simulink model "pendulotriple"  (R2023b)
settings: Solver=ode15s  StartTime=0.0  StopTime=20  RelTol=1e-3
values from neighbouring files (symbols this model uses):
  BL = 0.00223579    [ILCadaptable.m]    (also in parametros3.m)
  C1 = [1 0 0 0]    [ILCadaptable.m]    (also in parametros3.m = [1 0 0 0 0 0])
  C2 = [0 1 0 0]    [ILCadaptable.m]    (also in parametros3.m = [0 0 1 0 0 0])
  C3 = [0 0 1 0]    [ILCadaptable.m]    (also in parametros3.m = [0 0 0 0 1 0])
  Cv1 = [0 1 0 0 0 0]    [parametros3.m]
  Cv2 = [0 0 0 1 0 0]    [parametros3.m]
  Cv3 = [0 0 0 0 0 1]    [parametros3.m]
  ek1_1 = out.ek1    [ILCadaptable.m]    (also in parametros3.m)
  ek2_1 = out.ek2    [ILCadaptable.m]    (also in parametros3.m)
  ek3_1 = out.ek3    [parametros3.m]
  JL = 0.00040095    [ILCadaptable.m]    (also in parametros3.m)
  KB = 0.23351629    [ILCadaptable.m]    (also in parametros3.m)
  KM = 0.23351629    [ILCadaptable.m]    (also in parametros3.m)
  L1 = 2    [ILCadaptable.m]    (also in parametros3.m)
  L2 = 2    [ILCadaptable.m]    (also in parametros3.m)
  L3 = 2    [ILCadaptable.m]    (also in parametros3.m)
  LC = 0.0015    [ILCadaptable.m]    (also in parametros3.m)
  RC = 3.4    [ILCadaptable.m]    (also in parametros3.m)
  rt = 10    [ILCadaptable.m]    (also in parametros3.m)
libraries: slpidlib x3, simulink x3
settings Model: Creator=LENOVO  LastModifiedBy=LENOVO

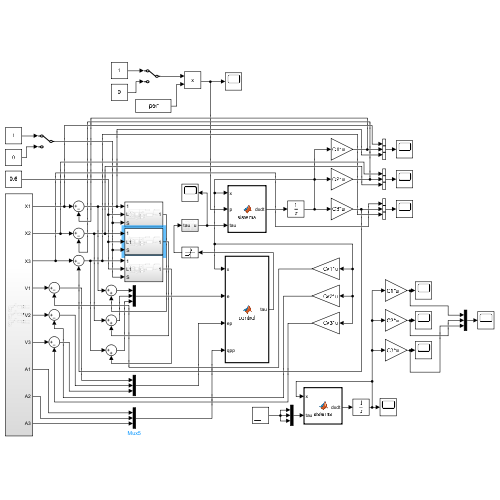
[thumbnail: Simulink's stored preview of the top-level diagram]
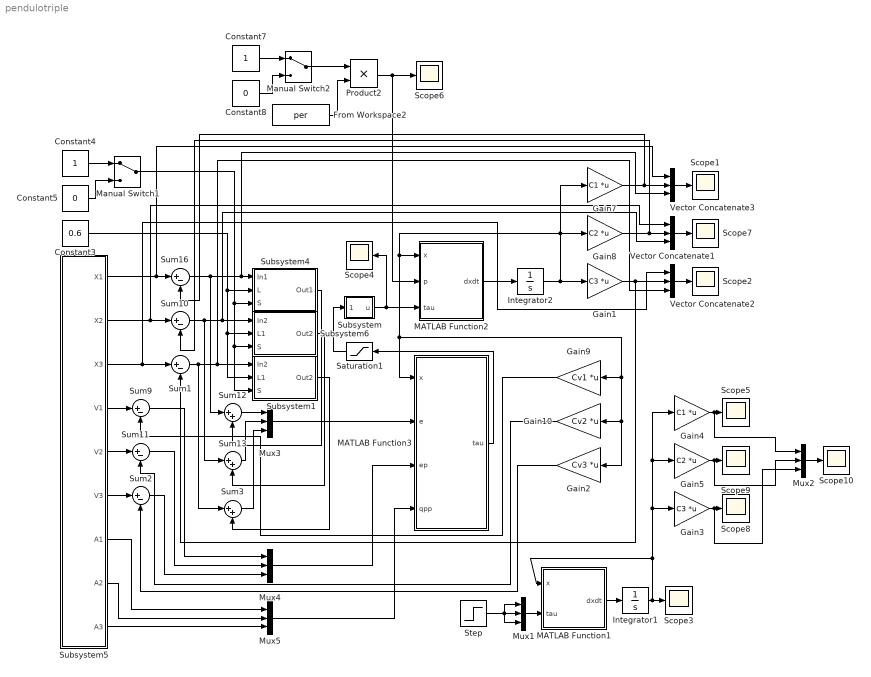
== system pendulotriple ==
  Constant3 : Constant  Value=0.6
  Constant4 : Constant
  Constant5 : Constant  Value=0
  Constant7 : Constant
  Constant8 : Constant  Value=0
  From Workspace2 : FromWorkspace  VariableName=per
  Gain1 : Gain  Gain=C3  Multiplication=Matrix(K*u)
  Gain10 : Gain  Gain=Cv2  Multiplication=Matrix(K*u)
  Gain2 : Gain  Gain=Cv3  Multiplication=Matrix(K*u)
  Gain3 : Gain  Gain=C3  Multiplication=Matrix(K*u)
  Gain4 : Gain  Gain=C1  Multiplication=Matrix(K*u)
  Gain5 : Gain  Gain=C2  Multiplication=Matrix(K*u)
  Gain7 : Gain  Gain=C1  Multiplication=Matrix(K*u)
  Gain8 : Gain  Gain=C2  Multiplication=Matrix(K*u)
  Gain9 : Gain  Gain=Cv1  Multiplication=Matrix(K*u)
  Integrator1 : Integrator  InitialCondition=[0 0 0 0 0 0]
  Integrator2 : Integrator  InitialCondition=[-pi/2 0 1 0 pi 0.1]
  MATLAB Function1 : MATLAB Function  TreatAsAtomicUnit=on
  MATLAB Function2 : MATLAB Function  TreatAsAtomicUnit=on
  MATLAB Function3 : MATLAB Function  TreatAsAtomicUnit=on
  Manual Switch1 : ManualSwitch
  Manual Switch2 : ManualSwitch
  Mux{1..5} (5 alike) : Mux  Inputs=3
  Product2 : Product
  Saturation1 : Saturate  UpperLimit=2  LowerLimit=-2
  Scope{1..10} (10 alike) : Scope
  Step : Step  Time=0  After=0  SampleTime=0
  Subsystem : Subsystem
  Subsystem1 : Subsystem
  Subsystem4 : Subsystem
  Subsystem5 : Subsystem
  Subsystem6 : Subsystem
  Sum{1..2,9..11,16} (6 alike) : Sum  Inputs=|+-
  Sum12 : Sum  Inputs=|++
  Sum13 : Sum  Inputs=|++
  Sum3 : Sum  Inputs=|++
  Vector Concatenate1 : Concatenate  NumInputs=3
  Vector Concatenate2 : Concatenate  NumInputs=3
  Vector Concatenate3 : Concatenate  NumInputs=3
  wires:
  MATLAB Function2/1(dxdt) -> Integrator2/1
  Subsystem/1(u) -> Scope4/1, MATLAB Function2/3(tau)
  Saturation1/1 -> Subsystem/1(tau)
  MATLAB Function3/1(tau) -> Saturation1/1
  Integrator2/1 -> Gain1/1, Gain7/1, Gain8/1, MATLAB Function2/1(x), Gain9/1, Gain2/1, Gain10/1, MATLAB Function3/1(x)
  Subsystem6/1(Out2) -> Sum13/2
  Subsystem5/7(A1) -> Mux5/1
  Sum13/1 -> Mux3/2
  Subsystem5/2(X2) -> Vector Concatenate1/1, Sum10/1
  Subsystem5/1(X1) -> Vector Concatenate3/1, Sum16/1
  Subsystem5/5(V2) -> Sum11/1
  Sum10/1 -> Sum13/1, Vector Concatenate1/3, Subsystem6/1(In2)
  Subsystem5/8(A2) -> Mux5/2
  Sum12/1 -> Mux3/1
  Sum16/1 -> Sum12/1, Vector Concatenate3/3, Subsystem4/1(In1)
  Constant3/1 -> Subsystem1/2(L1), Subsystem6/2(L1), Subsystem4/2(L)
  Sum11/1 -> Mux4/2
  Manual Switch1/1 -> Subsystem1/3(S), Subsystem6/3(S), Subsystem4/3(S)
  Subsystem5/4(V1) -> Sum9/1
  Subsystem4/1(Out1) -> Sum12/2
  Sum9/1 -> Mux4/1
  Constant4/1 -> Manual Switch1/1
  Constant5/1 -> Manual Switch1/2
  Subsystem5/3(X3) -> Vector Concatenate2/1, Sum1/1
  Sum1/1 -> Sum3/1, Vector Concatenate2/3, Subsystem1/1(In2)
  Subsystem5/6(V3) -> Sum2/1
  Mux3/1 -> MATLAB Function3/2(e)
  Sum3/1 -> Mux3/3
  Subsystem1/1(Out2) -> Sum3/2
  Sum2/1 -> Mux4/3
  Subsystem5/9(A3) -> Mux5/3
  Mux4/1 -> MATLAB Function3/3(ep)
  Mux5/1 -> MATLAB Function3/4(qpp)
  Gain9/1 -> Sum9/2
  Gain10/1 -> Sum11/2
  Gain2/1 -> Sum2/2
  Vector Concatenate1/1 -> Scope7/1
  Vector Concatenate3/1 -> Scope1/1
  Vector Concatenate2/1 -> Scope2/1
  Gain7/1 -> Sum16/2, Vector Concatenate3/2
  Gain8/1 -> Vector Concatenate1/2, Sum10/2
  Gain1/1 -> Sum1/2, Vector Concatenate2/2
  Product2/1 -> MATLAB Function2/2(p), Scope6/1
  Constant8/1 -> Manual Switch2/2
  Manual Switch2/1 -> Product2/1
  From Workspace2/1 -> Product2/2
  Constant7/1 -> Manual Switch2/1
  MATLAB Function1/1(dxdt) -> Integrator1/1
  Integrator1/1 -> MATLAB Function1/1(x), Gain3/1, Gain5/1, Gain4/1, Scope3/1
  Mux1/1 -> MATLAB Function1/2(tau)
  Step/1 -> Mux1/3, Mux1/1, Mux1/2
  Gain3/1 -> Mux2/3, Scope8/1
  Gain5/1 -> Mux2/2, Scope9/1
  Gain4/1 -> Mux2/1, Scope5/1
  Mux2/1 -> Scope10/1

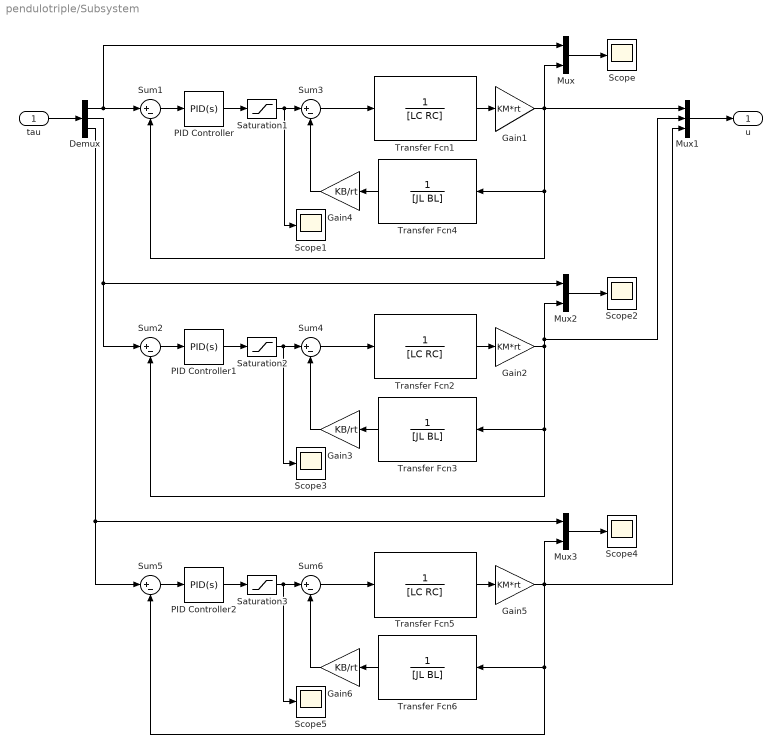
== system pendulotriple/Subsystem ==
  tau : Inport
  Demux : Demux  Outputs=3
  Gain1 : Gain  Gain=KM*rt
  Gain2 : Gain  Gain=KM*rt
  Gain3 : Gain  Gain=KB/rt
  Gain4 : Gain  Gain=KB/rt
  Gain5 : Gain  Gain=KM*rt
  Gain6 : Gain  Gain=KB/rt
  Mux : Mux  Inputs=2
  Mux1 : Mux  Inputs=3
  Mux2 : Mux  Inputs=2
  Mux3 : Mux  Inputs=2
  PID Controller : slpidlib/PID Controller  Controller=PID  Form=Parallel  TimeDomain=Continuous-time  UseExternalTs=off  SampleTime=-1  IntegratorMethod=Forward Euler  FilterMethod=Forward Euler  ControllerParametersSource=internal  P=100  I=50  UseKiTs=off  D=20  N=100  UseFilter=on  TunerSelectOption=Transfer Function Based (PID Tuner App)  InitialConditionSource=internal  InitialConditionForIntegrator=0  InitialConditionForFilter=0  DifferentiatorICPrevScaledInput=0  ExternalReset=none  TrackingMode=off  Kt=1  LimitOutput=off  SatLimitsSource=internal  UpperSaturationLimit=inf  LowerSaturationLimit=-inf  LinearizeAsGain=on  AntiWindupMode=none  Kb=1  LimitIntegrator=off  UpperIntegratorSaturationLimit=inf  LowerIntegratorSaturationLimit=-inf  POutMin=[]  POutMax=[]  IOutMin=[]  IOutMax=[]  DOutMin=[]  DOutMax=[]  NOutMin=[]  NOutMax=[]  SumOutMin=[]  SumOutMax=[]  SaturationOutMin=[]  SaturationOutMax=[]  PParamMin=[]  PParamMax=[]  IParamMin=[]  IParamMax=[]  DParamMin=[]  DParamMax=[]  NParamMin=[]  NParamMax=[]  KbParamMin=[]  KbParamMax=[]  KtParamMin=[]  KtParamMax=[]  KbOutMin=[]  KbOutMax=[]  KtOutMin=[]  KtOutMax=[]  IntegratorOutMin=[]  IntegratorOutMax=[]  FilterOutMin=[]  FilterOutMax=[]  SumI1OutMin=[]  SumI1OutMax=[]  SumI2OutMin=[]  SumI2OutMax=[]  SumI3OutMin=[]  SumI3OutMax=[]  SumI4OutMin=[]  SumI4OutMax=[]  SumDOutMin=[]  SumDOutMax=[]  DifferentiatorOutMin=[]  DifferentiatorOutMax=[]  FilterDiffOutCoefMin=[]  FilterDiffOutCoefMax=[]  ReciprocalOutMin=[]  ReciprocalOutMax=[]  SumDenOutMin=[]  SumDenOutMax=[]  SumNumOutMin=[]  SumNumOutMax=[]  DivideOutMin=[]  DivideOutMax=[]  UdiffTsProdOutMin=[]  UdiffTsProdOutMax=[]  NTsProdOutMin=[]  NTsProdOutMax=[]  UintegralTsProdOutMin=[]  UintegralTsProdOutMax=[]  UngainTsProdOutMin=[]  UngainTsProdOutMax=[]  ClampingZeroOutDataTypeStr=Inherit: Inherit via back propagation  ClampingZeroOutMin=[]  ClampingZeroOutMax=[]  FilterDenConstantOutDataTypeStr=Inherit: Inherit via back propagation  FilterDenConstantOutMin=[]  FilterDenConstantOutMax=[]  PCopyOutDataTypeStr=Inherit: Inherit via back propagation  PCopyOutMin=[]  PCopyOutMax=[]  NCopyOutDataTypeStr=Inherit: Inherit via back propagation  NCopyOutMin=[]  NCopyOutMax=[]  IntegratorContinuousStateAttributes=''  IntegratorStateMustResolveToSignalObject=off  IntegratorRTWStateStorageClass=Auto  FilterContinuousStateAttributes=''  FilterStateMustResolveToSignalObject=off  FilterRTWStateStorageClass=Auto  ParallelPVariant=InternalParameters  IdealPVariant=Disabled  IVariant=InternalParameters  DVariant=InternalParameters  IntegratorVariant=Continuous  SatVariant=Disabled  AWVariant=Passthrough  PCopyVariant=Disabled  TRVariant=Disabled  FdbkBlocksVariant=Forward  IdealPFdbkVariant=Disabled  SatFdbkVariant=Disabled  DerivativeFilterVariant=ContFilter  NVariant=InternalParameters  NCopyVariant=Disabled  FilterICVariant=InternalICsFilter  IntegratorICVariant=InternalICs  ExternalResetVariant=Disabled  TRSumVariant=Passthrough  SumFdbkVariant=Disabled  SumVariant=Sum_PID  TsampFilterVariant=InternalTs  TsampNgainVariant=Passthrough  TsampIntegralVariant=Disabled_SignalSpec  ExternalSaturationOutDataTypeStr=Inherit: Same as second input
  PID Controller1 : slpidlib/PID Controller  Controller=PID  Form=Parallel  TimeDomain=Continuous-time  UseExternalTs=off  SampleTime=-1  IntegratorMethod=Forward Euler  FilterMethod=Forward Euler  ControllerParametersSource=internal  P=100  I=50  UseKiTs=off  D=20  N=100  UseFilter=on  TunerSelectOption=Transfer Function Based (PID Tuner App)  InitialConditionSource=internal  InitialConditionForIntegrator=0  InitialConditionForFilter=0  DifferentiatorICPrevScaledInput=0  ExternalReset=none  TrackingMode=off  Kt=1  LimitOutput=off  SatLimitsSource=internal  UpperSaturationLimit=inf  LowerSaturationLimit=-inf  LinearizeAsGain=on  AntiWindupMode=none  Kb=1  LimitIntegrator=off  UpperIntegratorSaturationLimit=inf  LowerIntegratorSaturationLimit=-inf  POutMin=[]  POutMax=[]  IOutMin=[]  IOutMax=[]  DOutMin=[]  DOutMax=[]  NOutMin=[]  NOutMax=[]  SumOutMin=[]  SumOutMax=[]  SaturationOutMin=[]  SaturationOutMax=[]  PParamMin=[]  PParamMax=[]  IParamMin=[]  IParamMax=[]  DParamMin=[]  DParamMax=[]  NParamMin=[]  NParamMax=[]  KbParamMin=[]  KbParamMax=[]  KtParamMin=[]  KtParamMax=[]  KbOutMin=[]  KbOutMax=[]  KtOutMin=[]  KtOutMax=[]  IntegratorOutMin=[]  IntegratorOutMax=[]  FilterOutMin=[]  FilterOutMax=[]  SumI1OutMin=[]  SumI1OutMax=[]  SumI2OutMin=[]  SumI2OutMax=[]  SumI3OutMin=[]  SumI3OutMax=[]  SumI4OutMin=[]  SumI4OutMax=[]  SumDOutMin=[]  SumDOutMax=[]  DifferentiatorOutMin=[]  DifferentiatorOutMax=[]  FilterDiffOutCoefMin=[]  FilterDiffOutCoefMax=[]  ReciprocalOutMin=[]  ReciprocalOutMax=[]  SumDenOutMin=[]  SumDenOutMax=[]  SumNumOutMin=[]  SumNumOutMax=[]  DivideOutMin=[]  DivideOutMax=[]  UdiffTsProdOutMin=[]  UdiffTsProdOutMax=[]  NTsProdOutMin=[]  NTsProdOutMax=[]  UintegralTsProdOutMin=[]  UintegralTsProdOutMax=[]  UngainTsProdOutMin=[]  UngainTsProdOutMax=[]  ClampingZeroOutDataTypeStr=Inherit: Inherit via back propagation  ClampingZeroOutMin=[]  ClampingZeroOutMax=[]  FilterDenConstantOutDataTypeStr=Inherit: Inherit via back propagation  FilterDenConstantOutMin=[]  FilterDenConstantOutMax=[]  PCopyOutDataTypeStr=Inherit: Inherit via back propagation  PCopyOutMin=[]  PCopyOutMax=[]  NCopyOutDataTypeStr=Inherit: Inherit via back propagation  NCopyOutMin=[]  NCopyOutMax=[]  IntegratorContinuousStateAttributes=''  IntegratorStateMustResolveToSignalObject=off  IntegratorRTWStateStorageClass=Auto  FilterContinuousStateAttributes=''  FilterStateMustResolveToSignalObject=off  FilterRTWStateStorageClass=Auto  ParallelPVariant=InternalParameters  IdealPVariant=Disabled  IVariant=InternalParameters  DVariant=InternalParameters  IntegratorVariant=Continuous  SatVariant=Disabled  AWVariant=Passthrough  PCopyVariant=Disabled  TRVariant=Disabled  FdbkBlocksVariant=Forward  IdealPFdbkVariant=Disabled  SatFdbkVariant=Disabled  DerivativeFilterVariant=ContFilter  NVariant=InternalParameters  NCopyVariant=Disabled  FilterICVariant=InternalICsFilter  IntegratorICVariant=InternalICs  ExternalResetVariant=Disabled  TRSumVariant=Passthrough  SumFdbkVariant=Disabled  SumVariant=Sum_PID  TsampFilterVariant=InternalTs  TsampNgainVariant=Passthrough  TsampIntegralVariant=Disabled_SignalSpec  ExternalSaturationOutDataTypeStr=Inherit: Same as second input
  PID Controller2 : slpidlib/PID Controller  Controller=PID  Form=Parallel  TimeDomain=Continuous-time  UseExternalTs=off  SampleTime=-1  IntegratorMethod=Forward Euler  FilterMethod=Forward Euler  ControllerParametersSource=internal  P=100  I=50  UseKiTs=off  D=20  N=100  UseFilter=on  TunerSelectOption=Transfer Function Based (PID Tuner App)  InitialConditionSource=internal  InitialConditionForIntegrator=0  InitialConditionForFilter=0  DifferentiatorICPrevScaledInput=0  ExternalReset=none  TrackingMode=off  Kt=1  LimitOutput=off  SatLimitsSource=internal  UpperSaturationLimit=inf  LowerSaturationLimit=-inf  LinearizeAsGain=on  AntiWindupMode=none  Kb=1  LimitIntegrator=off  UpperIntegratorSaturationLimit=inf  LowerIntegratorSaturationLimit=-inf  POutMin=[]  POutMax=[]  IOutMin=[]  IOutMax=[]  DOutMin=[]  DOutMax=[]  NOutMin=[]  NOutMax=[]  SumOutMin=[]  SumOutMax=[]  SaturationOutMin=[]  SaturationOutMax=[]  PParamMin=[]  PParamMax=[]  IParamMin=[]  IParamMax=[]  DParamMin=[]  DParamMax=[]  NParamMin=[]  NParamMax=[]  KbParamMin=[]  KbParamMax=[]  KtParamMin=[]  KtParamMax=[]  KbOutMin=[]  KbOutMax=[]  KtOutMin=[]  KtOutMax=[]  IntegratorOutMin=[]  IntegratorOutMax=[]  FilterOutMin=[]  FilterOutMax=[]  SumI1OutMin=[]  SumI1OutMax=[]  SumI2OutMin=[]  SumI2OutMax=[]  SumI3OutMin=[]  SumI3OutMax=[]  SumI4OutMin=[]  SumI4OutMax=[]  SumDOutMin=[]  SumDOutMax=[]  DifferentiatorOutMin=[]  DifferentiatorOutMax=[]  FilterDiffOutCoefMin=[]  FilterDiffOutCoefMax=[]  ReciprocalOutMin=[]  ReciprocalOutMax=[]  SumDenOutMin=[]  SumDenOutMax=[]  SumNumOutMin=[]  SumNumOutMax=[]  DivideOutMin=[]  DivideOutMax=[]  UdiffTsProdOutMin=[]  UdiffTsProdOutMax=[]  NTsProdOutMin=[]  NTsProdOutMax=[]  UintegralTsProdOutMin=[]  UintegralTsProdOutMax=[]  UngainTsProdOutMin=[]  UngainTsProdOutMax=[]  ClampingZeroOutDataTypeStr=Inherit: Inherit via back propagation  ClampingZeroOutMin=[]  ClampingZeroOutMax=[]  FilterDenConstantOutDataTypeStr=Inherit: Inherit via back propagation  FilterDenConstantOutMin=[]  FilterDenConstantOutMax=[]  PCopyOutDataTypeStr=Inherit: Inherit via back propagation  PCopyOutMin=[]  PCopyOutMax=[]  NCopyOutDataTypeStr=Inherit: Inherit via back propagation  NCopyOutMin=[]  NCopyOutMax=[]  IntegratorContinuousStateAttributes=''  IntegratorStateMustResolveToSignalObject=off  IntegratorRTWStateStorageClass=Auto  FilterContinuousStateAttributes=''  FilterStateMustResolveToSignalObject=off  FilterRTWStateStorageClass=Auto  ParallelPVariant=InternalParameters  IdealPVariant=Disabled  IVariant=InternalParameters  DVariant=InternalParameters  IntegratorVariant=Continuous  SatVariant=Disabled  AWVariant=Passthrough  PCopyVariant=Disabled  TRVariant=Disabled  FdbkBlocksVariant=Forward  IdealPFdbkVariant=Disabled  SatFdbkVariant=Disabled  DerivativeFilterVariant=ContFilter  NVariant=InternalParameters  NCopyVariant=Disabled  FilterICVariant=InternalICsFilter  IntegratorICVariant=InternalICs  ExternalResetVariant=Disabled  TRSumVariant=Passthrough  SumFdbkVariant=Disabled  SumVariant=Sum_PID  TsampFilterVariant=InternalTs  TsampNgainVariant=Passthrough  TsampIntegralVariant=Disabled_SignalSpec  ExternalSaturationOutDataTypeStr=Inherit: Same as second input
  Saturation1 : Saturate  UpperLimit=250  LowerLimit=-250
  Saturation2 : Saturate  UpperLimit=250  LowerLimit=-250
  Saturation3 : Saturate  UpperLimit=250  LowerLimit=-250
  Scope{,1..5} (6 alike) : Scope
  Sum{1..6} (6 alike) : Sum  Inputs=|+-
  Transfer Fcn1 : TransferFcn  Denominator=[LC RC]
  Transfer Fcn2 : TransferFcn  Denominator=[LC RC]
  Transfer Fcn3 : TransferFcn  Denominator=[JL BL]
  Transfer Fcn4 : TransferFcn  Denominator=[JL BL]
  Transfer Fcn5 : TransferFcn  Denominator=[LC RC]
  Transfer Fcn6 : TransferFcn  Denominator=[JL BL]
  u : Outport
  wires:
  tau/1 -> Demux/1
  Demux/1 -> Sum1/1, Mux/1
  Mux/1 -> Scope/1
  Sum1/1 -> PID Controller/1
  Transfer Fcn1/1 -> Gain1/1
  Gain1/1 -> Sum1/2, Transfer Fcn4/1, Mux1/1, Mux/2
  Gain4/1 -> Sum3/2
  Sum3/1 -> Transfer Fcn1/1
  Transfer Fcn4/1 -> Gain4/1
  Mux1/1 -> u/1
  PID Controller/1 -> Saturation1/1
  PID Controller1/1 -> Saturation2/1
  Sum2/1 -> PID Controller1/1
  Demux/2 -> Sum2/1, Mux2/1
  Transfer Fcn2/1 -> Gain2/1
  Transfer Fcn3/1 -> Gain3/1
  Gain3/1 -> Sum4/2
  Gain2/1 -> Mux2/2, Mux1/2, Sum2/2, Transfer Fcn3/1
  Mux2/1 -> Scope2/1
  Sum4/1 -> Transfer Fcn2/1
  Saturation1/1 -> Scope1/1, Sum3/1
  Saturation2/1 -> Scope3/1, Sum4/1
  Mux3/1 -> Scope4/1
  Saturation3/1 -> Scope5/1, Sum6/1
  Sum6/1 -> Transfer Fcn5/1
  Transfer Fcn6/1 -> Gain6/1
  Transfer Fcn5/1 -> Gain5/1
  Demux/3 -> Mux3/1, Sum5/1
  Gain5/1 -> Mux1/3, Sum5/2, Transfer Fcn6/1, Mux3/2
  Sum5/1 -> PID Controller2/1
  Gain6/1 -> Sum6/2
  PID Controller2/1 -> Saturation3/1

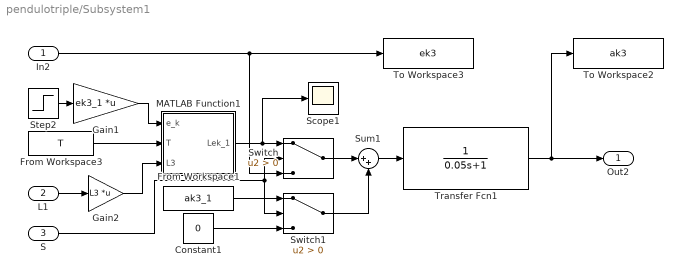
== system pendulotriple/Subsystem1 ==
  In2 : Inport
  L1 : Inport  Port=2
  S : Inport  Port=3
  Constant1 : Constant  Value=0
  From Workspace1 : FromWorkspace  VariableName=ak3_1
  From Workspace3 : FromWorkspace  VariableName=T
  Gain1 : Gain  Gain=ek3_1  Multiplication=Matrix(K*u)
  Gain2 : Gain  Gain=L3  Multiplication=Matrix(K*u)
  MATLAB Function1 : MATLAB Function  TreatAsAtomicUnit=on
  Scope1 : Scope
  Step2 : Step  Time=0  SampleTime=0
  Sum1 : Sum  Inputs=|++
  Switch : Switch  Criteria=u2 > Threshold  SaturateOnIntegerOverflow=off  InputSameDT=off
  Switch1 : Switch  Criteria=u2 > Threshold  SaturateOnIntegerOverflow=off  InputSameDT=off
  To Workspace2 : ToWorkspace  VariableName=ak3  SampleTime=-1
  To Workspace3 : ToWorkspace  VariableName=ek3  SampleTime=-1
  Transfer Fcn1 : TransferFcn  Denominator=[0.05 1]
  Out2 : Outport
  wires:
  MATLAB Function1/1(Lek_1) -> Scope1/1, Switch/1
  S/1 -> Switch1/2, Switch/2
  Sum1/1 -> Transfer Fcn1/1
  Gain1/1 -> MATLAB Function1/1(e_k)
  Transfer Fcn1/1 -> To Workspace2/1, Out2/1
  In2/1 -> Switch/3, To Workspace3/1
  From Workspace1/1 -> Switch1/1
  From Workspace3/1 -> MATLAB Function1/2(T)
  Constant1/1 -> Switch1/3
  Step2/1 -> Gain1/1
  Switch1/1 -> Sum1/2
  Switch/1 -> Sum1/1
  L1/1 -> Gain2/1
  Gain2/1 -> MATLAB Function1/3(L3)

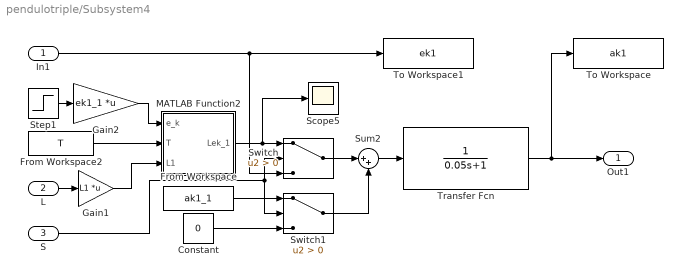
== system pendulotriple/Subsystem4 ==
  In1 : Inport
  L : Inport  Port=2
  S : Inport  Port=3
  Constant : Constant  Value=0
  From Workspace : FromWorkspace  VariableName=ak1_1
  From Workspace2 : FromWorkspace  VariableName=T
  Gain1 : Gain  Gain=L1  Multiplication=Matrix(K*u)
  Gain2 : Gain  Gain=ek1_1  Multiplication=Matrix(K*u)
  MATLAB Function2 : MATLAB Function  TreatAsAtomicUnit=on
  Scope5 : Scope
  Step1 : Step  Time=0  SampleTime=0
  Sum2 : Sum  Inputs=|++
  Switch : Switch  Criteria=u2 > Threshold  SaturateOnIntegerOverflow=off  InputSameDT=off
  Switch1 : Switch  Criteria=u2 > Threshold  SaturateOnIntegerOverflow=off  InputSameDT=off
  To Workspace : ToWorkspace  VariableName=ak1  SampleTime=-1
  To Workspace1 : ToWorkspace  VariableName=ek1  SampleTime=-1
  Transfer Fcn : TransferFcn  Denominator=[0.05 1]
  Out1 : Outport
  wires:
  From Workspace2/1 -> MATLAB Function2/2(T)
  In1/1 -> Switch/3, To Workspace1/1
  Gain2/1 -> MATLAB Function2/1(e_k)
  Step1/1 -> Gain2/1
  Constant/1 -> Switch1/3
  MATLAB Function2/1(Lek_1) -> Scope5/1, Switch/1
  Sum2/1 -> Transfer Fcn/1
  Switch1/1 -> Sum2/2
  From Workspace/1 -> Switch1/1
  Switch/1 -> Sum2/1
  Transfer Fcn/1 -> To Workspace/1, Out1/1
  L/1 -> Gain1/1
  S/1 -> Switch1/2, Switch/2
  Gain1/1 -> MATLAB Function2/3(L1)

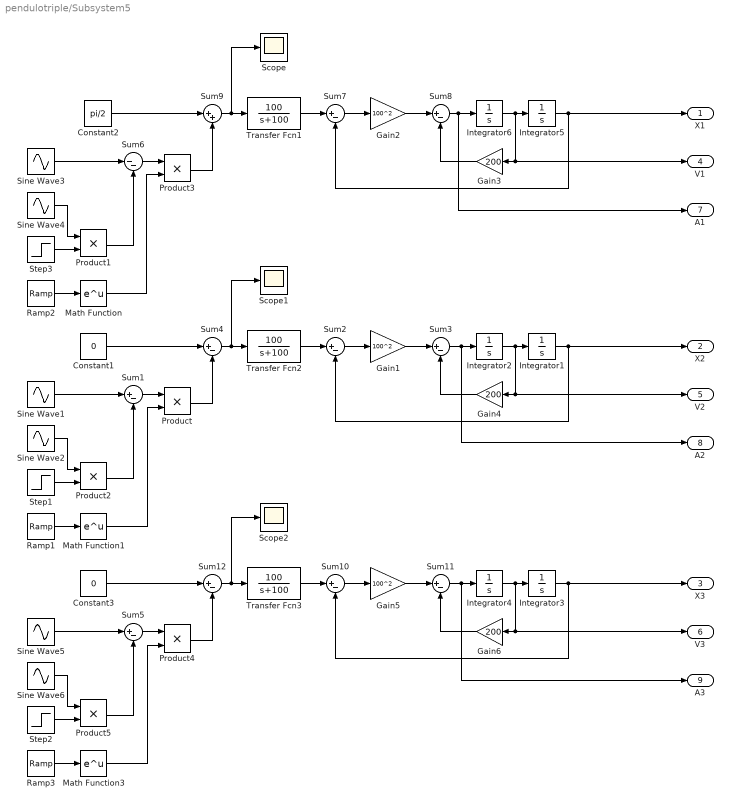
== system pendulotriple/Subsystem5 ==
  Constant1 : Constant  Value=0
  Constant2 : Constant  Value=pi/2
  Constant3 : Constant  Value=0
  Gain1 : Gain  Gain=100^2
  Gain2 : Gain  Gain=100^2
  Gain3 : Gain  Gain=200
  Gain4 : Gain  Gain=200
  Gain5 : Gain  Gain=100^2
  Gain6 : Gain  Gain=200
  Integrator{1..6} (6 alike) : Integrator
  Math Function : Math
  Math Function1 : Math
  Math Function3 : Math
  Product{,1..5} (6 alike) : Product
  Ramp1 : simulink/Sources/Ramp  slope=0  start=10  InitialOutput=0
  Ramp2 : simulink/Sources/Ramp  slope=0  start=10  InitialOutput=0
  Ramp3 : simulink/Sources/Ramp  slope=0  start=10  InitialOutput=0
  Scope : Scope
  Scope1 : Scope
  Scope2 : Scope
  Sine Wave{1..6} (6 alike) : Sin  Amplitude=2  Frequency=1.5  SampleTime=0
  Step1 : Step  Time=0  After=0  SampleTime=0
  Step2 : Step  Time=0  After=0  SampleTime=0
  Step3 : Step  Time=0  After=0  SampleTime=0
  Sum{1..5,7..8,10..12} (10 alike) : Sum  Inputs=|+-
  Sum6 : Sum  Inputs=|--
  Sum9 : Sum  Inputs=|++
  Transfer Fcn1 : TransferFcn  Numerator=[100]  Denominator=[1 100]
  Transfer Fcn2 : TransferFcn  Numerator=[100]  Denominator=[1 100]
  Transfer Fcn3 : TransferFcn  Numerator=[100]  Denominator=[1 100]
  X1 : Outport
  X2 : Outport  Port=2
  X3 : Outport  Port=3
  V1 : Outport  Port=4
  V2 : Outport  Port=5
  V3 : Outport  Port=6
  A1 : Outport  Port=7
  A2 : Outport  Port=8
  A3 : Outport  Port=9
  wires:
  Sine Wave3/1 -> Sum6/1
  Sum7/1 -> Gain2/1
  Sum8/1 -> A1/1, Integrator6/1
  Sine Wave4/1 -> Product1/1
  Gain2/1 -> Sum8/1
  Transfer Fcn1/1 -> Sum7/1
  Gain3/1 -> Sum8/2
  Product1/1 -> Sum6/2
  Step3/1 -> Product1/2
  Constant2/1 -> Sum9/1
  Integrator6/1 -> Gain3/1, V1/1, Integrator5/1
  Sum9/1 -> Scope/1, Transfer Fcn1/1
  Sum4/1 -> Scope1/1, Transfer Fcn2/1
  Sum3/1 -> A2/1, Integrator2/1
  Gain1/1 -> Sum3/1
  Transfer Fcn2/1 -> Sum2/1
  Sum2/1 -> Gain1/1
  Step1/1 -> Product2/2
  Constant1/1 -> Sum4/1
  Integrator1/1 -> X2/1, Sum2/2
  Sine Wave1/1 -> Sum1/1
  Gain4/1 -> Sum3/2
  Integrator2/1 -> V2/1, Gain4/1, Integrator1/1
  Product2/1 -> Sum1/2
  Sine Wave2/1 -> Product2/1
  Math Function/1 -> Product3/2
  Math Function1/1 -> Product/2
  Ramp2/1 -> Math Function/1
  Ramp1/1 -> Math Function1/1
  Sum6/1 -> Product3/1
  Product3/1 -> Sum9/2
  Sum1/1 -> Product/1
  Product/1 -> Sum4/2
  Integrator5/1 -> Sum7/2, X1/1
  Sine Wave6/1 -> Product5/1
  Transfer Fcn3/1 -> Sum10/1
  Integrator4/1 -> V3/1, Gain6/1, Integrator3/1
  Step2/1 -> Product5/2
  Gain6/1 -> Sum11/2
  Gain5/1 -> Sum11/1
  Sum12/1 -> Scope2/1, Transfer Fcn3/1
  Sum11/1 -> A3/1, Integrator4/1
  Sum5/1 -> Product4/1
  Constant3/1 -> Sum12/1
  Sum10/1 -> Gain5/1
  Product4/1 -> Sum12/2
  Ramp3/1 -> Math Function3/1
  Math Function3/1 -> Product4/2
  Integrator3/1 -> X3/1, Sum10/2
  Product5/1 -> Sum5/2
  Sine Wave5/1 -> Sum5/1

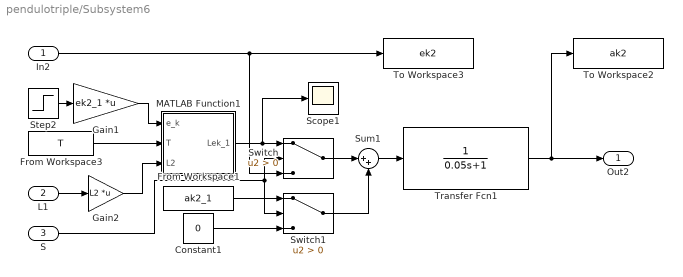
== system pendulotriple/Subsystem6 ==
  In2 : Inport
  L1 : Inport  Port=2
  S : Inport  Port=3
  Constant1 : Constant  Value=0
  From Workspace1 : FromWorkspace  VariableName=ak2_1
  From Workspace3 : FromWorkspace  VariableName=T
  Gain1 : Gain  Gain=ek2_1  Multiplication=Matrix(K*u)
  Gain2 : Gain  Gain=L2  Multiplication=Matrix(K*u)
  MATLAB Function1 : MATLAB Function  TreatAsAtomicUnit=on
  Scope1 : Scope
  Step2 : Step  Time=0  SampleTime=0
  Sum1 : Sum  Inputs=|++
  Switch : Switch  Criteria=u2 > Threshold  SaturateOnIntegerOverflow=off  InputSameDT=off
  Switch1 : Switch  Criteria=u2 > Threshold  SaturateOnIntegerOverflow=off  InputSameDT=off
  To Workspace2 : ToWorkspace  VariableName=ak2  SampleTime=-1
  To Workspace3 : ToWorkspace  VariableName=ek2  SampleTime=-1
  Transfer Fcn1 : TransferFcn  Denominator=[0.05 1]
  Out2 : Outport
  wires:
  MATLAB Function1/1(Lek_1) -> Scope1/1, Switch/1
  S/1 -> Switch1/2, Switch/2
  Sum1/1 -> Transfer Fcn1/1
  Gain1/1 -> MATLAB Function1/1(e_k)
  Transfer Fcn1/1 -> To Workspace2/1, Out2/1
  In2/1 -> Switch/3, To Workspace3/1
  From Workspace1/1 -> Switch1/1
  From Workspace3/1 -> MATLAB Function1/2(T)
  Constant1/1 -> Switch1/3
  Step2/1 -> Gain1/1
  Switch1/1 -> Sum1/2
  Switch/1 -> Sum1/1
  L1/1 -> Gain2/1
  Gain2/1 -> MATLAB Function1/3(L2)

== matlab function pendulotriple/Subsystem1/MATLAB Function1 ==
  data: Lek_1 output; e_k input; T input; L3 input
function Lek_1 = noncausal(e_k,T,L3)
n = int32(T);
Lek_1 = L3*(e_k(n+1) - e_k(n))/0.03;

== matlab function pendulotriple/MATLAB Function1 ==
  data: x input; tau input; dxdt output
function dxdt = sistema(x,tau)

%definición de parametros
m1 = 0.066;
m2 = 0.0792;
m3 = 0.0792;
l1 = 0.25;
l2 = 0.3;
l3 = 0.3;
lc1 = l1/2;
lc2 = l2/2;
lc3 = l3/2;
I1 = 0.00138;
I2 = 0.00238;
I3 = 0.00338;
b = 0.1;
g = 9.81;

%calculo de las constantes del sistema
a1 = m1*lc1^2+(m2+m3)*l1^2+I1;
a2 = m2*lc2^2+m3*l2^2+I2;
a3 = m3*lc3^2+I3;
a4 = m2*l1*lc2+m3*l1*l2;
a5 = m3*l1*lc3;
a6 = m3*l2*lc3;
a7 = m1*lc1+(m2+m3)*l1;
a8 = m2*lc2+m3*l2;
a9 = m3*lc3;

%variables de estado
x1 = x(1);
x2 = x(2);
x3 = x(3);
x4 = x(4);
x5 = x(5);
x6 = x(6);

%Matrices del sistema
G1 = a7*cos(x1)+a8*cos(x1+x3)+a9*cos(x1+x3+x5);
G2 = a8*cos(x1+x3)+a9*cos(x1+x3+x5);
G3 = a9*cos(x1+x3+x5);
G = g*[G1;G2;G3];%matriz de gravedad 

C11 = 0; C22 = C11; C33 = C11;
C12 = -2*(a4*sin(x3)+a5*sin(x3+x5))*x2-(a4*sin(x3)+a5*sin(x3+x5))*x4-a5*sin(x3+x5)*x6;
C21 = -(a4*sin(x3)+a5*sin(x3+x5))*x2+a5*sin(x3+x5)*x6;
C13 = -2*(a5*sin(x3+x5)+a6*sin(x5))*x2-(a5*sin(x3+x5)+2*a6*sin(x5))*x4-(a5*sin(x3+x5)+a6*sin(x5))*x6;
C31 = (a5*sin(x3+x5)+a6*sin(x5))*x2+(a5*sin(x3+x5)+2*a6*sin(x5))*x4;
C23 = -(a5*sin(x3+x5)+2*a6*sin(x5))*x2-2*a6*sin(x5)*x4-a5*sin(x5)*x6;
C32 = -a5*sin(x3+x5)*x2+a6*sin(x5)*x4;
C = [C11,C12,C13;
    C21,C22,C23;
    C31,C32,C33];%matriz de velocidad o coriolis

M11 = a1+a2+a3+2*a4*cos(x3)+2*a5*cos(x3+x5)+2*a6*cos(x5);
M22 = a2+a3+2*a6*cos(x5);
M33 = a3;
M12 = a2+a3+a4*cos(x3)+a5*cos(x3+x5)+2*a6*cos(x5); M21 = M12;
M23 = a3+a5*cos(x5); M32 = M23;
M13 = a3+a5*cos(x3+x5)+a6*cos(x5); M31=M13;
M = [M11,M12,M13;
    M21,M22,M23;
    M31,M32,M33];%matriz de aceleración

%d/dt[x1;x2;x3;x4;x5;x6]=[f1;f2;f3;f4;f5;f6]
%calculo de f2 y f4 
u = tau - b*[x2;x4;x6];
xb = M^(-1)*u-M^(-1)*C*[x2;x4;x6]-M^(-1)*G;

%sistema en la forma d/dt[x1;x2;x3;x4;x5;x6]=[f1;f2;f3;f4;f5;f6]
dxdt = [x2; 
        xb(1);
        x4;
        xb(2);
        x6;
        xb(3)];

== matlab function pendulotriple/MATLAB Function2 ==
  data: x input; p input; tau input; dxdt output
function dxdt = sistema(x,p,tau)

%definición de parametros
m1 = 0.066;
m2 = 0.0792;
m3 = 0.0792;
l1 = 0.25;
l2 = 0.3;
l3 = 0.3;
lc1 = l1/2;
lc2 = l2/2;
lc3 = l3/2;
I1 = 0.00138;
I2 = 0.00238;
I3 = 0.00338;
b = 0.1;
g = 9.81;

%calculo de las constantes del sistema
a1 = m1*lc1^2+(m2+m3)*l1^2+I1;
a2 = m2*lc2^2+m3*l2^2+I2;
a3 = m3*lc3^2+I3;
a4 = m2*l1*lc2+m3*l1*l2;
a5 = m3*l1*lc3;
a6 = m3*l2*lc3;
a7 = m1*lc1+(m2+m3)*l1;
a8 = m2*lc2+m3*l2;
a9 = m3*lc3;

%Perturbación paramétrica
a1=a1+p(1);
a2=a2+p(2);
a3=a3+p(3);
a4=a4+p(4);
a5=a5+p(5);
a6=a6+p(6);
a7=a7+p(7);
a8=a8+p(8);
a9=a9+p(9);

%variables de estado
x1 = x(1);
x2 = x(2);
x3 = x(3);
x4 = x(4);
x5 = x(5);
x6 = x(6);

%Matrices del sistema
G1 = a7*cos(x1)+a8*cos(x1+x3)+a9*cos(x1+x3+x5);
G2 = a8*cos(x1+x3)+a9*cos(x1+x3+x5);
G3 = a9*cos(x1+x3+x5);
G = g*[G1;G2;G3];%matriz de gravedad 

C11 = 0; C22 = C11; C33 = C11;
C12 = -2*(a4*sin(x3)+a5*sin(x3+x5))*x2-(a4*sin(x3)+a5*sin(x3+x5))*x4-a5*sin(x3+x5)*x6;
C21 = -(a4*sin(x3)+a5*sin(x3+x5))*x2+a5*sin(x3+x5)*x6;
C13 = -2*(a5*sin(x3+x5)+a6*sin(x5))*x2-(a5*sin(x3+x5)+2*a6*sin(x5))*x4-(a5*sin(x3+x5)+a6*sin(x5))*x6;
C31 = (a5*sin(x3+x5)+a6*sin(x5))*x2+(a5*sin(x3+x5)+2*a6*sin(x5))*x4;
C23 = -(a5*sin(x3+x5)+2*a6*sin(x5))*x2-2*a6*sin(x5)*x4-a5*sin(x5)*x6;
C32 = -a5*sin(x3+x5)*x2+a6*sin(x5)*x4;
C = [C11,C12,C13;
    C21,C22,C23;
    C31,C32,C33];%matriz de velocidad o coriolis

M11 = a1+a2+a3+2*a4*cos(x3)+2*a5*cos(x3+x5)+2*a6*cos(x5);
M22 = a2+a3+2*a6*cos(x5);
M33 = a3;
M12 = a2+a3+a4*cos(x3)+a5*cos(x3+x5)+2*a6*cos(x5); M21 = M12;
M23 = a3+a5*cos(x5); M32 = M23;
M13 = a3+a5*cos(x3+x5)+a6*cos(x5); M31=M13;
M = [M11,M12,M13;
    M21,M22,M23;
    M31,M32,M33];%matriz de aceleración

%d/dt[x1;x2;x3;x4;x5;x6]=[f1;f2;f3;f4;f5;f6]
%calculo de f2 y f4 
u = tau - b*[x2;x4;x6];
xb = M^(-1)*u-M^(-1)*C*[x2;x4;x6]-M^(-1)*G;

%sistema en la forma d/dt[x1;x2;x3;x4;x5;x6]=[f1;f2;f3;f4;f5;f6]
dxdt = [x2; 
        xb(1);
        x4;
        xb(2);
        x6;
        xb(3)];

== matlab function pendulotriple/MATLAB Function3 ==
  data: x input; e input; ep input; qpp input; tau output
function tau = control(x,e,ep,qpp)

%constantes del controlador
kp = 40;
kv = 20;

%definición de parametros
m1 = 0.066;
m2 = 0.0792;
m3 = 0.0792;
l1 = 0.25;
l2 = 0.3;
l3 = 0.3;
lc1 = l1/2;
lc2 = l2/2;
lc3 = l3/2;
I1 = 0.00138;
I2 = 0.00238;
I3 = 0.00338;
b = 0.1;
g = 9.81;

%calculo de las constantes del sistema
a1 = m1*lc1^2+(m2+m3)*l1^2+I1;
a2 = m2*lc2^2+m3*l2^2+I2;
a3 = m3*lc3^2+I3;
a4 = m2*l1*lc2+m3*l1*l2;
a5 = m3*l1*lc3;
a6 = m3*l2*lc3;
a7 = m1*lc1+(m2+m3)*l1;
a8 = m2*lc2+m3*l2;
a9 = m3*lc3;

%variables de estado
x1 = x(1);
x2 = x(2);
x3 = x(3);
x4 = x(4);
x5 = x(5);
x6 = x(6);

%Matrices del sistema
G1 = a7*cos(x1)+a8*cos(x1+x3)+a9*cos(x1+x3+x5);
G2 = a8*cos(x1+x3)+a9*cos(x1+x3+x5);
G3 = a9*cos(x1+x3+x5);
G = g*[G1;G2;G3];%matriz de gravedad 

C11 = 0; C22 = C11; C33 = C11;
C12 = -2*(a4*sin(x3)+a5*sin(x3+x5))*x2-(a4*sin(x3)+a5*sin(x3+x5))*x4-a5*sin(x3+x5)*x6;
C21 = -(a4*sin(x3)+a5*sin(x3+x5))*x2+a5*sin(x3+x5)*x6;
C13 = -2*(a5*sin(x3+x5)+a6*sin(x5))*x2-(a5*sin(x3+x5)+2*a6*sin(x5))*x4-(a5*sin(x3+x5)+a6*sin(x5))*x6;
C31 = (a5*sin(x3+x5)+a6*sin(x5))*x2+(a5*sin(x3+x5)+2*a6*sin(x5))*x4;
C23 = -(a5*sin(x3+x5)+2*a6*sin(x5))*x2-2*a6*sin(x5)*x4-a5*sin(x5)*x6;
C32 = -a5*sin(x3+x5)*x2+a6*sin(x5)*x4;
C = [C11,C12,C13;
    C21,C22,C23;
    C31,C32,C33];%matriz de velocidad o coriolis

M11 = a1+a2+a3+2*a4*cos(x3)+2*a5*cos(x3+x5)+2*a6*cos(x5);
M22 = a2+a3+2*a6*cos(x5);
M33 = a3;
M12 = a2+a3+a4*cos(x3)+a5*cos(x3+x5)+2*a6*cos(x5); M21 = M12;
M23 = a3+a5*cos(x5); M32 = M23;
M13 = a3+a5*cos(x3+x5)+a6*cos(x5); M31=M13;
M = [M11,M12,M13;
    M21,M22,M23;
    M31,M32,M33];%matriz de aceleración

%calculo de accion de control
tau = M*(qpp+kp*e+kv*ep)+C*[x2;x4;x6]+G+b*[x2;x4;x6];

== matlab function pendulotriple/Subsystem4/MATLAB Function2 ==
  data: Lek_1 output; e_k input; T input; L1 input
function Lek_1 = noncausal(e_k,T,L1)
n = int32(T);
Lek_1 = L1*(e_k(n+1) - e_k(n))/0.03;

== matlab function pendulotriple/Subsystem6/MATLAB Function1 ==
  data: Lek_1 output; e_k input; T input; L2 input
function Lek_1 = noncausal(e_k,T,L2)
n = int32(T);
Lek_1 = L2*(e_k(n+1) - e_k(n))/0.03;
